simulink model "ACC_Decision_SPPVT_Integrated"  (R2024b)
settings: Solver=FixedStepAuto  StartTime=0.0  StopTime=0.05  FixedStep=0.05  RelTol=1e-3  EnableMultiTasking=on
settings Model: Creator=ZhaoY  LastModifiedBy=ZhaoY
settings SolverCC: AutoInsertRateTranBlk=on
settings DataIOCC: ExternalInput=input_data  LoadExternalInput=on

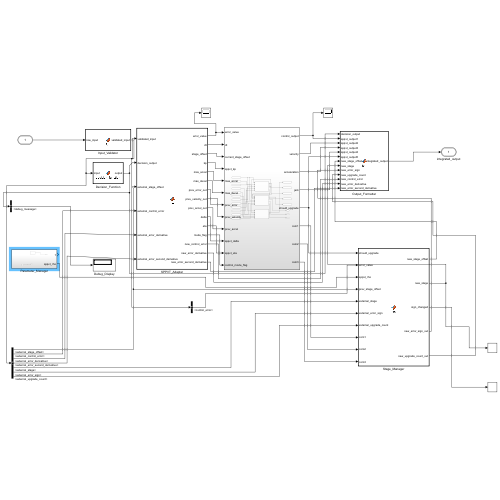
[thumbnail: Simulink's stored preview of the top-level diagram]
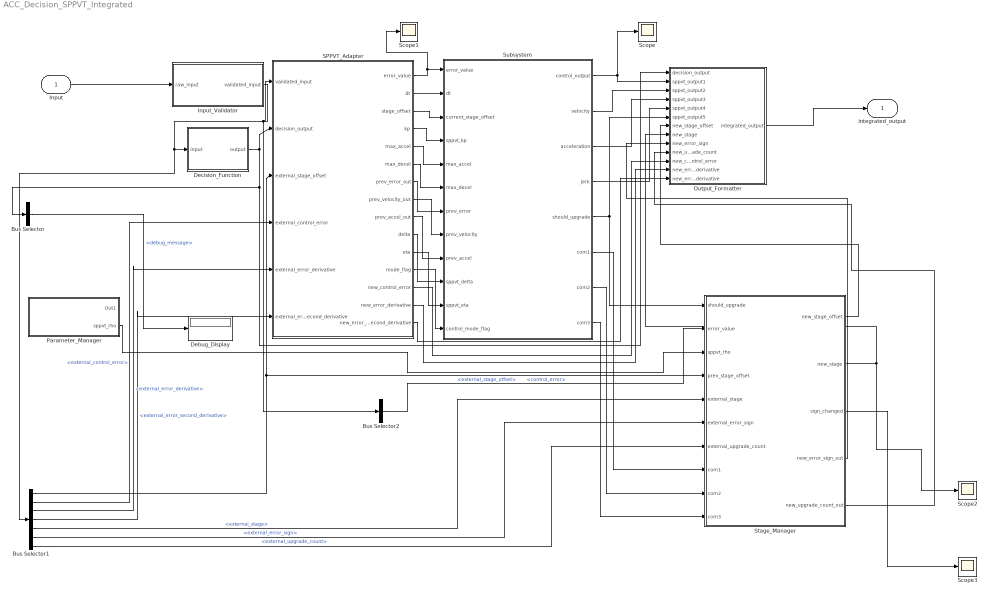
== system ACC_Decision_SPPVT_Integrated ==
  Input : Inport  OutDataTypeStr=Bus: DecisionSPPVTInputExtended  PortDimensions=1
  Bus Selector : BusSelector  OutputSignals=debug_message
  Bus Selector1 : BusSelector  OutputSignals=external_stage_offset,external_control_error,external_error_derivative,external_error_second_derivative,external_stage,external_error_sign,external_upgrade_count
  Bus Selector2 : BusSelector  OutputSignals=control_error
  Debug_Display : Display
  Decision_Function : MATLAB Function  TreatAsAtomicUnit=on
  Input_Validator : MATLAB Function  TreatAsAtomicUnit=on
  Output_Formatter : MATLAB Function  TreatAsAtomicUnit=on
  Parameter_Manager : Subsystem
  SPPVT_Adapter : MATLAB Function  TreatAsAtomicUnit=on
  Scope{,1..3} (4 alike) : Scope
  Stage_Manager : MATLAB Function  TreatAsAtomicUnit=on
  Subsystem : Subsystem
  integrated_output : Outport  OutDataTypeStr=Bus: DecisionSPPVTOutputExtended
  wires:
  Input/1 -> Input_Validator/1(raw_input)
  Input_Validator/1(validated_input) -> Bus Selector2/1, SPPVT_Adapter/1(validated_input), Bus Selector1/1, Decision_Function/1(input)
  Decision_Function/1(output) -> Output_Formatter/1(decision_output), Bus Selector/1, SPPVT_Adapter/2(decision_output)
  SPPVT_Adapter/1(error_value) -> Subsystem/1(error_value), Scope1/1
  Output_Formatter/1(integrated_output) -> integrated_output/1
  Bus Selector/1 -> Debug_Display/1  "<debug_message>"
  Stage_Manager/2(new_stage) -> Scope2/1, Output_Formatter/8(new_stage)
  Stage_Manager/3(sign_changed) -> Scope3/1
  Parameter_Manager/2(sppvt_rho) -> Stage_Manager/3(sppvt_rho)
  Bus Selector1/1 -> SPPVT_Adapter/3(external_stage_offset), Stage_Manager/4(prev_stage_offset)  "<external_stage_offset>"
  Bus Selector2/1 -> Stage_Manager/2(error_value)  "<control_error>"
  Stage_Manager/1(new_stage_offset) -> Output_Formatter/7(new_stage_offset)
  Subsystem/1(control_output) -> Output_Formatter/2(sppvt_output1), Scope/1
  Subsystem/5(should_upgrade) -> Stage_Manager/1(should_upgrade), Output_Formatter/6(sppvt_output5)
  SPPVT_Adapter/2(dt) -> Subsystem/2(dt)
  SPPVT_Adapter/3(stage_offset) -> Subsystem/3(current_stage_offset)
  SPPVT_Adapter/4(kp) -> Subsystem/4(sppvt_kp)
  SPPVT_Adapter/5(max_accel) -> Subsystem/5(max_accel)
  SPPVT_Adapter/6(max_decel) -> Subsystem/6(max_decel)
  SPPVT_Adapter/7(prev_error_out) -> Subsystem/7(prev_error)
  SPPVT_Adapter/8(prev_velocity_out) -> Subsystem/8(prev_velocity)
  SPPVT_Adapter/9(prev_accel_out) -> Subsystem/9(prev_accel)
  SPPVT_Adapter/10(delta) -> Subsystem/10(sppvt_delta)
  SPPVT_Adapter/11(eta) -> Subsystem/11(sppvt_eta)
  SPPVT_Adapter/12(mode_flag) -> Subsystem/12(control_mode_flag)
  Subsystem/2(velocity) -> Output_Formatter/3(sppvt_output2)
  Subsystem/3(acceleration) -> Output_Formatter/4(sppvt_output3)
  Subsystem/4(jerk) -> Output_Formatter/5(sppvt_output4)
  Subsystem/6(com1) -> Stage_Manager/8(com1)
  Subsystem/7(com2) -> Stage_Manager/9(com2)
  Subsystem/8(com3) -> Stage_Manager/10(com3)
  Bus Selector1/2 -> SPPVT_Adapter/4(external_control_error)  "<external_control_error>"
  Bus Selector1/3 -> SPPVT_Adapter/5(external_error_derivative)  "<external_error_derivative>"
  Bus Selector1/4 -> SPPVT_Adapter/6(external_error_second_derivative)  "<external_error_second_derivative>"
  SPPVT_Adapter/13(new_control_error) -> Output_Formatter/11(new_control_error)
  SPPVT_Adapter/14(new_error_derivative) -> Output_Formatter/12(new_error_derivative)
  SPPVT_Adapter/15(new_error_second_derivative) -> Output_Formatter/13(new_error_second_derivative)
  Bus Selector1/5 -> Stage_Manager/5(external_stage)  "<external_stage>"
  Bus Selector1/6 -> Stage_Manager/6(external_error_sign)  "<external_error_sign>"
  Bus Selector1/7 -> Stage_Manager/7(external_upgrade_count)  "<external_upgrade_count>"
  Stage_Manager/5(new_upgrade_count_out) -> Output_Formatter/10(new_upgrade_count)
  Stage_Manager/4(new_error_sign_out) -> Output_Formatter/9(new_error_sign)

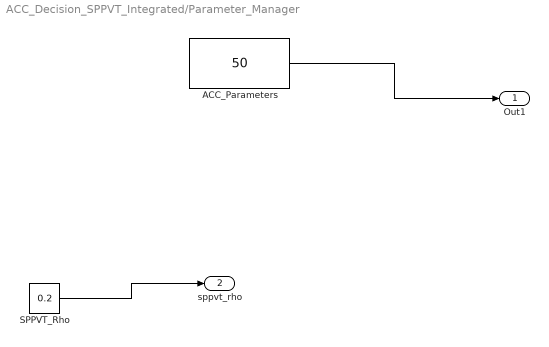
== system ACC_Decision_SPPVT_Integrated/Parameter_Manager ==
  ACC_Parameters : Constant  Value=50
  SPPVT_Rho : Constant  Value=0.2
  Out1 : Outport
  sppvt_rho : Outport  Port=2
  wires:
  ACC_Parameters/1 -> Out1/1
  SPPVT_Rho/1 -> sppvt_rho/1

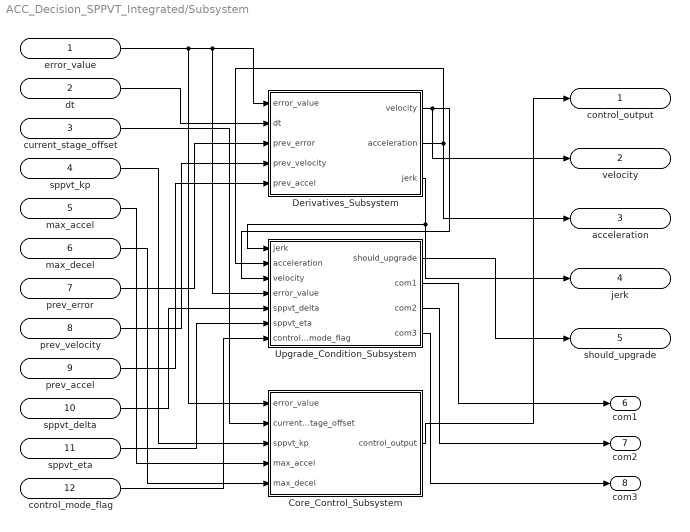
== system ACC_Decision_SPPVT_Integrated/Subsystem ==
  error_value : Inport
  dt : Inport  Port=2
  current_stage_offset : Inport  Port=3
  sppvt_kp : Inport  Port=4
  max_accel : Inport  Port=5
  max_decel : Inport  Port=6
  prev_error : Inport  Port=7
  prev_velocity : Inport  Port=8
  prev_accel : Inport  Port=9
  sppvt_delta : Inport  Port=10
  sppvt_eta : Inport  Port=11
  control_mode_flag : Inport  Port=12
  Core_Control_Subsystem : Subsystem
  Derivatives_Subsystem : Subsystem
  Upgrade_Condition_Subsystem : Subsystem
  control_output : Outport
  velocity : Outport  Port=2
  acceleration : Outport  Port=3
  jerk : Outport  Port=4
  should_upgrade : Outport  Port=5
  com1 : Outport  Port=6
  com2 : Outport  Port=7
  com3 : Outport  Port=8
  wires:
  Upgrade_Condition_Subsystem/1(should_upgrade) -> should_upgrade/1
  Derivatives_Subsystem/3(jerk) -> jerk/1, Upgrade_Condition_Subsystem/1(jerk)
  Derivatives_Subsystem/1(velocity) -> velocity/1, Upgrade_Condition_Subsystem/3(velocity)
  sppvt_eta/1 -> Upgrade_Condition_Subsystem/6(sppvt_eta)
  control_mode_flag/1 -> Upgrade_Condition_Subsystem/7(control_mode_flag)
  sppvt_delta/1 -> Upgrade_Condition_Subsystem/5(sppvt_delta)
  Derivatives_Subsystem/2(acceleration) -> acceleration/1, Upgrade_Condition_Subsystem/2(acceleration)
  Upgrade_Condition_Subsystem/2(com1) -> com1/1
  Upgrade_Condition_Subsystem/3(com2) -> com2/1
  Upgrade_Condition_Subsystem/4(com3) -> com3/1
  Core_Control_Subsystem/1(control_output) -> control_output/1
  max_decel/1 -> Core_Control_Subsystem/5(max_decel)
  max_accel/1 -> Core_Control_Subsystem/4(max_accel)
  sppvt_kp/1 -> Core_Control_Subsystem/3(sppvt_kp)
  current_stage_offset/1 -> Core_Control_Subsystem/2(current_stage_offset)
  prev_error/1 -> Derivatives_Subsystem/3(prev_error)
  prev_velocity/1 -> Derivatives_Subsystem/4(prev_velocity)
  prev_accel/1 -> Derivatives_Subsystem/5(prev_accel)
  dt/1 -> Derivatives_Subsystem/2(dt)
  error_value/1 -> Upgrade_Condition_Subsystem/4(error_value), Derivatives_Subsystem/1(error_value), Core_Control_Subsystem/1(error_value)

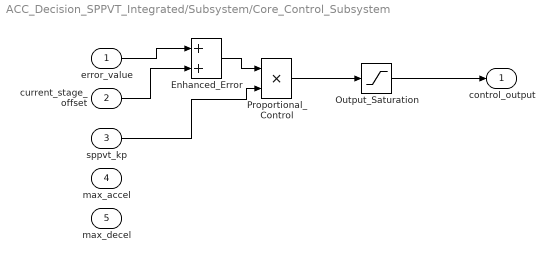
== system ACC_Decision_SPPVT_Integrated/Subsystem/Core_Control_Subsystem ==
  error_value : Inport
  current_stage_offset : Inport  Port=2
  sppvt_kp : Inport  Port=3
  max_accel : Inport  Port=4
  max_decel : Inport  Port=5
  Enhanced_Error : Sum
  Output_Saturation : Saturate  UpperLimit=2.0  LowerLimit=-3.0
  Proportional_Control : Product
  control_output : Outport
  wires:
  Proportional_Control/1 -> Output_Saturation/1
  Output_Saturation/1 -> control_output/1
  sppvt_kp/1 -> Proportional_Control/2
  current_stage_offset/1 -> Enhanced_Error/2
  error_value/1 -> Enhanced_Error/1
  Enhanced_Error/1 -> Proportional_Control/1

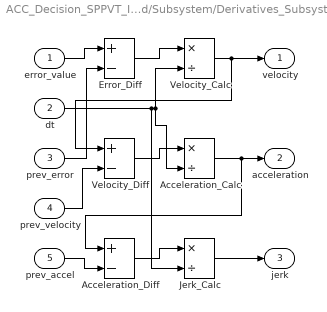
== system ACC_Decision_SPPVT_Integrated/Subsystem/Derivatives_Subsystem ==
  error_value : Inport
  dt : Inport  Port=2
  prev_error : Inport  Port=3
  prev_velocity : Inport  Port=4
  prev_accel : Inport  Port=5
  Acceleration_Calc : Product  Inputs=*/
  Acceleration_Diff : Sum  Inputs=+-
  Error_Diff : Sum  Inputs=+-
  Jerk_Calc : Product  Inputs=*/
  Velocity_Calc : Product  Inputs=*/
  Velocity_Diff : Sum  Inputs=+-
  velocity : Outport
  acceleration : Outport  Port=2
  jerk : Outport  Port=3
  wires:
  Velocity_Calc/1 -> Velocity_Diff/1, velocity/1
  Acceleration_Calc/1 -> Acceleration_Diff/1, acceleration/1
  Jerk_Calc/1 -> jerk/1
  error_value/1 -> Error_Diff/1
  prev_error/1 -> Error_Diff/2
  Error_Diff/1 -> Velocity_Calc/1
  prev_accel/1 -> Acceleration_Diff/2
  prev_velocity/1 -> Velocity_Diff/2
  Acceleration_Diff/1 -> Jerk_Calc/1
  dt/1 -> Jerk_Calc/2, Acceleration_Calc/2, Velocity_Calc/2
  Velocity_Diff/1 -> Acceleration_Calc/1

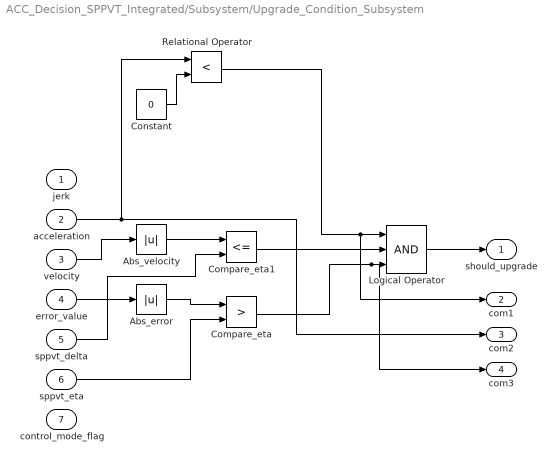
== system ACC_Decision_SPPVT_Integrated/Subsystem/Upgrade_Condition_Subsystem ==
  jerk : Inport
  acceleration : Inport  Port=2
  velocity : Inport  Port=3
  error_value : Inport  Port=4
  sppvt_delta : Inport  Port=5
  sppvt_eta : Inport  Port=6
  control_mode_flag : Inport  Port=7
  Abs_error : Abs  SaturateOnIntegerOverflow=off
  Abs_velocity : Abs  SaturateOnIntegerOverflow=off
  Compare_eta : RelationalOperator  Operator=>  OutDataTypeStr=boolean  RndMeth=Simplest  InputSameDT=off
  Compare_eta1 : RelationalOperator  Operator=<=  OutDataTypeStr=boolean  RndMeth=Simplest  InputSameDT=off
  Constant : Constant  Value=0
  Logical Operator : Logic  Inputs=3  AllPortsSameDT=off  OutDataTypeStr=boolean
  Relational Operator : RelationalOperator  Operator=<  OutDataTypeStr=boolean  RndMeth=Simplest  InputSameDT=off
  should_upgrade : Outport
  com1 : Outport  Port=2
  com2 : Outport  Port=3
  com3 : Outport  Port=4
  wires:
  error_value/1 -> Abs_error/1
  Abs_error/1 -> Compare_eta/1
  sppvt_eta/1 -> Compare_eta/2
  acceleration/1 -> com2/1, Relational Operator/1
  Constant/1 -> Relational Operator/2
  velocity/1 -> Abs_velocity/1
  Abs_velocity/1 -> Compare_eta1/1
  sppvt_delta/1 -> Compare_eta1/2
  Relational Operator/1 -> com1/1, Logical Operator/1
  Compare_eta1/1 -> Logical Operator/2
  Compare_eta/1 -> com3/1, Logical Operator/3
  Logical Operator/1 -> should_upgrade/1

== matlab function ACC_Decision_SPPVT_Integrated/Stage_Manager ==
  data: new_stage_offset output; should_upgrade input; new_stage output; sign_changed output; new_error_sign_out output; error_value input; sppvt_rho input; prev_stage_offset input; external_stage input; external_error_sign input; external_upgrade_count input; com1 input; com2 input; com3 input; new_upgrade_count_out output
  function [new_stage_offset, new_stage, sign_changed, new_error_sign_out, new_upgrade_count_out] = fcn(should_upgrade, error_value, sppvt_rho, prev_stage_offset, external_stage, external_error_sign, external_upgrade_count, com1, com2, com3)
  %#codegen
  % Stateless SPPVT Stage Manager with scalar-based state management
  % Compatible with 21/22-field bus design (all scalar version)

  % Extract states from input scalars (replaces persistent variables and array extraction)
  current_stage = int32(external_stage);
  prev_error_sign = int32(external_error_sign);
  upgrade_count = int32(external_upgrade_count);

  current_stage_offset = prev_stage_offset;

  % Calculate current error sign
  if abs(error_value) < 1e-6
      current_sign = int32(0);     % Near zero
  elseif error_value > 0
      current_sign = int32(1);     % Positive error
  else
      current_sign = int32(-1);    % Negative error
  end

  % Initialize outputs with current values
  new_stage = current_stage;
  sign_changed = false;

  % Error sign change detection
  if (prev_error_sign ~= 0) && (current_sign ~= 0) && (prev_error_sign ~= current_sign)
      % Sign change: reset to initial stage
      sign_changed = true;

      % Reset all states to initial level
      new_stage = int32(1);
      new_stage_offset = 0.0;      % Initial stage offset is 0
      upgrade_count = int32(0);

  elseif should_upgrade && ~sign_changed
      % No sign change and upgrade condition met
      new_stage = new_stage + int32(1);
      upgrade_count = upgrade_count + int32(1);

      % Calculate new stage offset based on error sign (consistent with existing logic)
      if error_value > 0
          % Positive error: increase positive stage offset
          new_stage_offset = prev_stage_offset + sppvt_rho * abs(error_value);
      else
          % Negative error: increase negative stage offset
          new_stage_offset = prev_stage_offset - sppvt_rho * abs(error_value);
      end

      % Limit stage offset range [-100, 100] to prevent infinite accumulation
      new_stage_offset = max(-100.0, min(100.0, new_stage_offset));

  else
      % No upgrade: maintain current state
      new_stage_offset = prev_stage_offset;
  end

  % Update error sign history (only for non-zero errors)
  new_error_sign = prev_error_sign;
  if current_sign ~= 0
      new_error_sign = current_sign;
  end

  % Output individual scalars for next cycle (to be captured by Python)
  % Scalar outputs: new_error_sign_out, new_upgrade_count_out (new_stage already in output list)
  new_error_sign_out = double(new_error_sign);
  new_upgrade_count_out = double(upgrade_count);

  % Print the three conditional variables using fprintf
  % Print the three conditional variables as 'true' or 'false' with detailed labels
  fprintf('Condition 1 (com1): %s\n', string(com1));
  fprintf('Condition 2 (com2): %f\n', double(com2));
  fprintf('Condition 3 (com3): %s\n', string(com3));
  end

== matlab function ACC_Decision_SPPVT_Integrated/Decision_Function ==
  data: input input Bus: DecisionSPPVTInputExtended; output output Bus: DecisionSPPVTOutputExtended
function output = decision_function(input)
%DECISION_FUNCTION ACC决策状态机的MATLAB实现
%   适用于MATLAB 2024b，在Simulink中作为MATLAB Function块使用
%   
%   输入: DecisionSPPVTInput总线
%   输出: 决策相关的输出结构
%
%   状态定义 (根据decision.md和acc_decision.py):
%   S0 = 0: 在控状态 (ACTIVE_CONTROL)
%   S1 = 1: 适速有史待命 (ADAPTIVE_HISTORY_STANDBY)  
% %   S2 = 2: 适速无史待命 (ADAPTIVE_NO_HISTORY_STANDBY)
%   S3 = 3: 低速状态 (LOW_SPEED)
%
%   决策定义:
%   R1 = 1: 速度降低 (DECREASE_SPEED)
%   R2 = 2: 速度增加 (INCREASE_SPEED)
%   R3 = 3: 时距降低 (DECREASE_DISTANCE)
%   R4 = 4: 时距增加 (INCREASE_DISTANCE)
%   R5 = 5: 无继控制 (ACTIVATE_CURRENT_SPEED)
%   R6 = 6: 继承控制 (ACTIVATE_INHERITED_SPEED)
%   R7 = 7: 扭矩仲裁 (TORQUE_ARBITRATION)
%   R8 = 8: 系统待命 (SYSTEM_STANDBY)

% 保留必要的persistent变量（仅用于调试计数）
persistent debug_counter

% 初始化调试计数器
if isempty(debug_counter)
    debug_counter = int32(0);
end

% 提取输入参数
ego_speed_kmh = input.ego_speed_kmh;
% ego_speed_ms = input.ego_speed_ms;          % 未使用，决策逻辑只需要km/h
command_type = input.command_type;
command_active = input.command_active;
manual_throttle_active = input.manual_throttle_active;
% control_error = input.control_error;        % 决策模块不直接使用控制误差
% control_mode_flag = input.control_mode_flag; % 决策模块不直接使用模式标志
input_V_target_kmh = input.V_target_kmh;
input_V_min_kmh = input.V_min_kmh;
input_G2_s = input.G2_s;
% timestamp = input.timestamp;                % 决策逻辑不需要时间戳

% 更新参数
V_target_kmh = input_V_target_kmh;
V_min_kmh = input_V_min_kmh;
G2_s = input_G2_s;

%% 键盘参数修改逻辑 (在状态机逻辑之前处理)
if command_active
    speed_step = 5.0;  % 速度调整步长 (km/h)
    time_gap_step = 0.2; % 时距调整步长 (s)

    switch command_type
        case 1 % I0: Decrease speed -> E key
            V_target_kmh = max(V_min_kmh, V_target_kmh - speed_step);
            fprintf('Keyboard: E key decrease speed, V_target: %.1f km/h\n', V_target_kmh);

        case 2 % I1: Increase speed -> Q key
            V_target_kmh = min(120.0, V_target_kmh + speed_step);
            fprintf('Keyboard: Q key increase speed, V_target: %.1f km/h\n', V_target_kmh);

        case 3 % I2: Decrease time gap -> T key
            G2_s = max(1.0, G2_s - time_gap_step);
            fprintf('Keyboard: T key decrease gap, G2: %.1f s\n', G2_s);

        case 4 % I3: Increase time gap -> R key
            G2_s = min(5.0, G2_s + time_gap_step);
            fprintf('Keyboard: R key increase gap, G2: %.1f s\n', G2_s);

        case 7 % I6: Cancel ACC -> C key
            fprintf('Keyboard: C key cancel ACC\n');
            % 取消逻辑在状态机中处理
    end
end

% 增加调试计数器
debug_counter = debug_counter + 1;

%% 从输入获取决策状态信息（替代persistent变量）
% 如果总线中没有这些字段，使用默认值
if isfield(input, 'current_state')
    current_state = input.current_state;
else
    current_state = int32(2); % 默认S2状态
end

if isfield(input, 'has_history')
    has_history = input.has_history;
else
    has_history = false; % 默认无历史
end

if isfield(input, 'last_active_decision')
    last_active_decision = input.last_active_decision;
else
    last_active_decision = int32(8); % 默认R8
end

%% 获取SPPVT状态外化字段（虽然决策模块不直接使用，但需要传递）
% 这些字段将在输出中保持原值，由SPPVT模块使用
if isfield(input, 'external_stage_offset')
    external_stage_offset = input.external_stage_offset;
else
    external_stage_offset = 0.0; % 默认级差
end

if isfield(input, 'external_stage')
    external_stage = input.external_stage;
else
    external_stage = 1.0; % 默认阶段
end

if isfield(input, 'external_error_sign')
    external_error_sign = input.external_error_sign;
else
    external_error_sign = 0.0; % 默认误差符号
end

if isfield(input, 'external_upgrade_count')
    external_upgrade_count = input.external_upgrade_count;
else
    external_upgrade_count = 0.0; % 默认升级计数
end

if isfield(input, 'external_control_error')
    external_control_error = input.external_control_error;
else
    external_control_error = 0.0; % 默认控制误差
end

if isfield(input, 'external_error_derivative')
    external_error_derivative = input.external_error_derivative;
else
    external_error_derivative = 0.0; % 默认控制误差导数
end

if isfield(input, 'external_error_second_derivative')
    external_error_second_derivative = input.external_error_second_derivative;
else
    external_error_second_derivative = 0.0; % 默认控制误差二阶导数
end

%% 状态机主逻辑 - 使用next_state管理状态转移
next_state = current_state; % 默认保持当前状态
next_has_history = has_history; % 默认保持历史状态
next_last_active_decision = last_active_decision; % 默认保持决策
torque_arbitration_active = false;

% 基于当前状态设置默认决策
if current_state == 0
    control_enabled = true;
    current_decision = last_active_decision; % 使用上次有效决策实现持续性
    % 如果历史决策无效，提供后备值
    if ~(current_decision >= 1 && current_decision <= 7)
        current_decision = int32(5); % 默认 R5: 无继控制
    end
else
    control_enabled = false;
    current_decision = int32(8); % R8: 系统待命
end

% 基于车速的自动状态转移
if ego_speed_kmh < V_min_kmh
    if current_state ~= 3
        next_state = int32(3); % 转移到S3: 低速状态
        control_enabled = false;
        current_decision = int32(8);
    end
else
    % 从S3状态恢复
    if current_state == 3
        if has_history
            next_state = int32(1); % 恢复到S1: 有史待命
        else
            next_state = int32(2); % 恢复到S2: 无史待命
        end
        control_enabled = false;
        current_decision = int32(8);
    end
end

% 处理激活的指令
if command_active
    switch current_state
        case 0 % S0: 在控状态
            [next_state, current_decision, control_enabled, torque_arbitration_active] = ...
                handle_active_control_state(command_type, ego_speed_kmh, manual_throttle_active, V_target_kmh, G2_s);

        case 1 % S1: 适速有史待命
            [next_state, current_decision, control_enabled, next_has_history, V_target_kmh, G2_s] = ...
                handle_adaptive_history_standby_state(command_type, ego_speed_kmh, V_target_kmh, G2_s, input_V_target_kmh, input_G2_s);

        case 2 % S2: 适速无史待命
            [next_state, current_decision, control_enabled, next_has_history, V_target_kmh, G2_s] = ...
                handle_adaptive_no_history_standby_state(command_type, ego_speed_kmh, input_V_target_kmh, input_G2_s);

        case 3 % S3: 低速状态
            % 低速状态下，指令不进入控制
            current_decision = int32(8);
            control_enabled = false;

        otherwise
            % 错误状态，重置到无史待命
            next_state = int32(2);
            current_decision = int32(8);
            control_enabled = false;
            next_has_history = false;
    end
end

% 更新有效决策用于持续性控制
if current_decision >= 1 && current_decision <= 7
    next_last_active_decision = current_decision;
end

%% 计算调试信息值（在赋值前准备）
control_flag = int32(control_enabled);
if mod(debug_counter, 20) == 0 % 每20个周期输出一次调试信息
    % 调试代码: 1000 + 状态*100 + 决策*10 + 控制使能标志
    debug_code = int32(1000 + current_state*100 + current_decision*10 + control_flag);
    debug_message_value = debug_code;

    % 添加MATLAB Function调试输出
    fprintf('Decision Function Debug: State=%d->%d, Decision=%d, Control=%d, Active=%d, Cmd=%d, DebugCode=%d\n', ...
            current_state, next_state, current_decision, int32(control_enabled), int32(command_active), command_type, debug_code);
else
    % 非调试周期显示简单计数器
    debug_message_value = debug_counter;
end

%% 构造输出 - 严格按照DecisionSPPVTOutputExtended总线定义顺序赋值所有22个字段
output = struct();

% 1-6: 来自决策系统的基本信息
output.control_enabled = logical(control_enabled);
output.current_state = int32(next_state);  % 修正：输出当前步计算的实际状态
output.current_decision = int32(current_decision);
output.torque_arbitration_active = logical(torque_arbitration_active);
output.updated_V_target_kmh = double(V_target_kmh);
output.updated_G2_s = double(G2_s);

% 7-11: SPPVT相关字段的默认值（这些将由后续模块填充）
output.sppvt_control_output = 0.0;
output.sppvt_velocity_output = 0.0;
output.sppvt_acceleration_output = 0.0;
output.sppvt_stage_output = 0.0;
output.sppvt_status_output = 0.0;

% 12: 调试信息
output.debug_message = debug_message_value;

% 13-15: 决策状态输出字段（状态外化支持）
output.next_state = int32(next_state);
output.next_has_history = logical(next_has_history);
output.next_last_active_decision = int32(next_last_active_decision);

% 16-22: SPPVT状态输出字段（传递外部输入，由后续SPPVT模块更新）- 全部标量化
output.new_stage_offset = double(external_stage_offset);
output.new_stage = double(external_stage);
output.new_error_sign = double(external_error_sign);
output.new_upgrade_count = double(external_upgrade_count);
output.new_control_error = double(external_control_error);
output.new_error_derivative = double(external_error_derivative);
output.new_error_second_derivative = double(external_error_second_derivative);

end

%% 状态处理函数

function [new_state, decision, control_enabled, torque_arbitration] = ...
    handle_active_control_state(command_type, ego_speed_kmh, manual_throttle_active, V_target_kmh, G2_s)
%处理在控状态 S0 (根据decision.md)

new_state = int32(0); % 默认保持在控状态
control_enabled = true;
torque_arbitration = false;

% 初始化所有输出变量（确保在所有执行路径上都有定义）
decision = int32(8); % 默认系统待命

switch command_type
    case 1 % I0: 降速指令
        decision = int32(1); % R1: 速度降低
        
    case 2 % I1: 增速指令
        decision = int32(2); % R2: 速度增加
        
    case 3 % I2: 降距指令
        decision = int32(3); % R3: 时距降低
        
    case 4 % I3: 增距指令
        decision = int32(4); % R4: 时距增加
        
    case 5 % I4: 油门指令
        decision = int32(7); % R7: 扭矩仲裁
        torque_arbitration = true;
        % 状态保持S0，但控制权可能被驾驶员超越
        
    case 6 % I5: 刹车指令
        new_state = int32(1); % 转到S1: 适速有史待命
        decision = int32(8); % R8: 系统待命
        control_enabled = false;
        
    case 7 % I6: 取消ACC指令
        new_state = int32(1); % 转到S1: 适速有史待命
        decision = int32(8); % R8: 系统待命
        control_enabled = false;
        
    otherwise
        decision = int32(8); % R8: 系统待命
end
end

function [new_state, decision, control_enabled, has_history, V_target_kmh, G2_s] = ...
    handle_adaptive_history_standby_state(command_type, ego_speed_kmh, current_V_target, current_G2, input_V_target, input_G2)
%处理适速有史待命状态 S1 (根据decision.md)

new_state = int32(1); % 默认保持S1状态
control_enabled = false;
has_history = true; % 保持历史数据

% 初始化所有输出变量（确保在所有执行路径上都有定义）
V_target_kmh = current_V_target;
G2_s = current_G2;
decision = int32(8); % 默认系统待命

switch command_type
    case 1 % I0: 降速指令
        new_state = int32(0); % 转到S0: 在控状态
        decision = int32(5); % R5: 无继控制 (当速启控)
        control_enabled = true;
        V_target_kmh = input_V_target; % 使用当前速度作为目标
        G2_s = input_G2;
        
    case 2 % I1: 增速指令
        new_state = int32(0); % 转到S0: 在控状态
        decision = int32(6); % R6: 继承控制 (使用历史速度)
        control_enabled = true;
        % V_target_kmh和G2_s保持历史值不变
        
    otherwise % I2-I6: 其他指令
        decision = int32(8); % R8: 系统待命
        % 状态保持S1，参数保持历史值
end
end

function [new_state, decision, control_enabled, has_history, V_target_kmh, G2_s] = ...
    handle_adaptive_no_history_standby_state(command_type, ego_speed_kmh, input_V_target, input_G2)
%处理适速无史待命状态 S2 (根据decision.md)

new_state = int32(2); % 默认保持S2状态
control_enabled = false;
has_history = false; % 仍然无历史数据

% 初始化所有输出变量（确保在所有执行路径上都有定义）
V_target_kmh = input_V_target;
G2_s = input_G2;
decision = int32(8); % 默认系统待命

switch command_type
    case 1 % I0: 降速指令
        new_state = int32(0); % 转到S0: 在控状态
        decision = int32(5); % R5: 无继控制 (当速启控)
        control_enabled = true;
        has_history = true; % 启控后产生历史数据
        V_target_kmh = input_V_target; % 使用当前速度作为目标
        G2_s = input_G2;
        
    otherwise % I1-I6: 其他指令
        decision = int32(8); % R8: 系统待命
        % 状态保持S2，无历史数据
        % V_target_kmh和G2_s已在函数开头初始化
end
end

== matlab function ACC_Decision_SPPVT_Integrated/Input_Validator ==
  data: raw_input input Bus: DecisionSPPVTInputExtended; validated_input output Bus: DecisionSPPVTInputExtended
function validated_input = fcn(raw_input)
%#codegen
%
% 输入验证和预处理
% 输入: raw_input (DecisionSPPVTInput总线)
% 输出: validated_input (经过验证和修正的总线)

validated_input = raw_input;

% 接下来，在输出变量上执行数值范围检查，防止异常值进入下游模块。
validated_input.ego_speed_kmh = max(0, min(200, raw_input.ego_speed_kmh));
validated_input.ego_speed_ms = max(0, min(60, raw_input.ego_speed_ms));
validated_input.V_target_kmh = max(30, min(120, raw_input.V_target_kmh));
validated_input.V_min_kmh = max(20, min(50, raw_input.V_min_kmh));
validated_input.G2_s = max(1.0, min(8.0, raw_input.G2_s));


% 确保最低车速始终小于或等于目标车速。
if validated_input.V_min_kmh > validated_input.V_target_kmh
    validated_input.V_min_kmh = validated_input.V_target_kmh - 10;
end

% 时间戳直接透传
validated_input.timestamp = raw_input.timestamp;

end

== matlab function ACC_Decision_SPPVT_Integrated/Output_Formatter ==
  data: decision_output input; integrated_output output Bus: DecisionSPPVTOutputExtended; sppvt_output1 input; sppvt_output2 input; sppvt_output3 input; sppvt_output4 input; sppvt_output5 input; new_stage_offset input; new_stage input; new_error_sign input; new_upgrade_count input; new_control_error input; new_error_derivative input; new_error_second_derivative input
function integrated_output = fcn(decision_output, sppvt_output1, sppvt_output2, sppvt_output3, sppvt_output4, sppvt_output5, new_stage_offset, new_stage, new_error_sign, new_upgrade_count, new_control_error, new_error_derivative, new_error_second_derivative)
%#codegen
% Output_Formatter - 21/22-field state externalization version (all scalar)
% Integrates decision, SPPVT output and state output for Python state capture
%
% Inputs:
%   decision_output - DecisionSPPVTOutput from Decision_Function (includes next_state and other decision state output fields)
%   sppvt_output1-5 - 5 outputs from SPPVT_Control (control, velocity, acceleration, jerk, status)
%   new_stage_offset - Stage offset (scalar)
%   new_stage - Stage Manager new stage (scalar)
%   new_error_sign - Stage Manager new error sign (scalar)
%   new_upgrade_count - Stage Manager new upgrade count (scalar)
%   new_control_error - New control error (scalar)
%   new_error_derivative - New control error derivative (scalar)
%   new_error_second_derivative - New control error second derivative (scalar)
%
% Output: integrated_output - DecisionSPPVTOutputExtended (22 fields)

%% 构造集成输出结构
integrated_output = struct();

%% 按照总线定义顺序赋值所有字段（确保代码生成兼容性）
% 根据DecisionSPPVTOutputExtended总线定义的22字段顺序

% 1-6: 来自决策系统的信息
integrated_output.control_enabled = decision_output.control_enabled;
integrated_output.current_state = decision_output.current_state;
integrated_output.current_decision = decision_output.current_decision;
integrated_output.torque_arbitration_active = decision_output.torque_arbitration_active;
integrated_output.updated_V_target_kmh = decision_output.updated_V_target_kmh;
integrated_output.updated_G2_s = decision_output.updated_G2_s;

% 7-11: SPPVT controller outputs (double precision)
integrated_output.sppvt_control_output = double(sppvt_output1);
integrated_output.sppvt_velocity_output = double(sppvt_output2);
integrated_output.sppvt_acceleration_output = double(sppvt_output3);
% 注意：sppvt_output4是jerk，不是stage，stage来自Stage_Manager
integrated_output.sppvt_stage_output = double(new_stage);  % 从Stage_Manager获取stage值（标量）
integrated_output.sppvt_status_output = double(sppvt_output5);

% 12: Debug information (composite code)
debug_code = int32(3000 + decision_output.current_state*100 + ...
                 mod(int32(sppvt_output5), 10)*10 + ...
                 int32(decision_output.control_enabled));
integrated_output.debug_message = debug_code;

% 13-15: Decision module state outputs
integrated_output.next_state = decision_output.next_state;
integrated_output.next_has_history = decision_output.next_has_history;
integrated_output.next_last_active_decision = decision_output.next_last_active_decision;

% 16-22: SPPVT state outputs consumed in Python (全部标量化)

% 16: Stage offset (scalar)
integrated_output.new_stage_offset = double(new_stage_offset);

% 17-19: Stage Manager states (全部标量)
integrated_output.new_stage = double(new_stage);
integrated_output.new_error_sign = double(new_error_sign);
integrated_output.new_upgrade_count = double(new_upgrade_count);

% 20-22: Adapter states - 控制误差及其导数 (全部标量)
% 修正：用SPPVT实际计算的导数值替换Adapter传来的占位值
integrated_output.new_control_error = double(new_control_error);
integrated_output.new_error_derivative = double(sppvt_output2);  % 误差的一阶导数 (velocity)
integrated_output.new_error_second_derivative = double(sppvt_output3);  % 误差的二阶导数 (acceleration)

% 调试输出（22字段版本，包含完整状态外化信息）
if mod(decision_output.debug_message, 50) == 0
    fprintf("Output_Formatter Input: State=%d, Decision=%d, Control=%d, Debug=%d\n", ...
            int32(decision_output.current_state), int32(decision_output.current_decision), ...
            int32(decision_output.control_enabled), int32(decision_output.debug_message));
    fprintf("Integrated Output: State=S%d->S%d, Decision=R%d, Control=%d, SPPVT=%.3f\n", ...
            int32(decision_output.current_state), int32(decision_output.next_state), ...
            int32(decision_output.current_decision), int32(decision_output.control_enabled), double(sppvt_output1));

    % 决策状态外化调试输出
    fprintf("Decision State: next_state=S%d, next_history=%d, next_decision=R%d\n", ...
            int32(decision_output.next_state), int32(decision_output.next_has_history), ...
            int32(decision_output.next_last_active_decision));

    % SPPVT状态外化调试输出（标量版本）
    fprintf("SPPVT State: StageOffset=%.3f, Stage=%.0f, ErrorSign=%.0f, UpgradeCount=%.0f\n", ...
            double(new_stage_offset), double(new_stage), double(new_error_sign), double(new_upgrade_count));
    fprintf("Error States: ControlError=%.3f, Derivative=%.3f, SecondDerivative=%.3f\n", ...
            double(new_control_error), double(sppvt_output2), double(sppvt_output3));
end

end

== matlab function ACC_Decision_SPPVT_Integrated/SPPVT_Adapter ==
  data: validated_input input; decision_output input; error_value output; dt output; stage_offset output; kp output; max_accel output; max_decel output; prev_error_out output; prev_velocity_out output; prev_accel_out output; delta output; eta output; mode_flag output; external_stage_offset input; external_control_error input; new_control_error output double; external_error_derivative input; external_error_second_derivative input; new_error_derivative output; new_error_second_derivative output
function [error_value, dt, stage_offset, kp, max_accel, max_decel, prev_error_out, prev_velocity_out, prev_accel_out, delta, eta, mode_flag, new_control_error, new_error_derivative, new_error_second_derivative] = fcn(validated_input, decision_output, external_stage_offset, external_control_error, external_error_derivative, external_error_second_derivative)
%#codegen
% SPPVT接口适配器 - 支持外部状态注入版本 (全部标量化)
% 输入:
%   validated_input - 验证后的输入总线
%   decision_output - 决策输出总线
%   external_stage_offset - 外部级差状态
%   external_control_error - 外部控制误差
%   external_error_derivative - 外部控制误差的导数
%   external_error_second_derivative - 外部控制误差的二阶导数
% 输出:
%   1-12: 12个独立信号匹配sppvt_control_model的12个输入端口
%   13-15: 新的误差状态（标量化）- new_control_error, new_error_derivative, new_error_second_derivative

%% 直接使用外部状态（从Bus Selector传入）- 全部标量化
current_stage_offset = external_stage_offset;

% 直接使用输入的标量参数（不再需要从数组提取）
% 注意：velocity和accel实际上是误差的一阶和二阶导数
prev_error = external_control_error;
prev_velocity = external_error_derivative;           % 控制误差的一阶导数
prev_accel = external_error_second_derivative;       % 控制误差的二阶导数

%% 根据决策结果确定控制误差
if decision_output.control_enabled
    % 控制激活时使用实际误差
    error_value = validated_input.control_error;
else
    % 控制未激活时误差为0
    error_value = 0.0;
end

%% 分配12个独立输出信号
dt = 0.05;                                      % [2] dt 时间步长 (硬编码为50ms)
stage_offset = current_stage_offset;            % [3] 当前级差 (状态变量)
kp = 1.0;                                       % [4] sppvt_kp 比例系数 (硬编码)
max_accel = 2.0;                                % [5] max_accel 最大加速度 (硬编码)
max_decel = -3.0;                               % [6] max_decel 最大减速度 (硬编码)
prev_error_out = prev_error;                    % [7] 上次误差 (状态变量)
prev_velocity_out = prev_velocity;              % [8] 上次速度 (状态变量)
prev_accel_out = prev_accel;                    % [9] 上次加速度 (状态变量)
delta = 0.05;                                   % [10] sppvt_delta 控制参数 
eta = 0.5;                                      % [11] sppvt_eta 控制参数 
mode_flag = double(validated_input.control_mode_flag); % [12] 控制模式标志

%% 输出新的误差状态（第13-15个输出）- 全部标量化
% 用于Output_Formatter的误差状态字段
% 注意：这些是当前计算的误差值，导数将由SPPVT模块计算
new_control_error = error_value;
new_error_derivative = external_error_derivative;  % 保持输入值，将由SPPVT更新
new_error_second_derivative = external_error_second_derivative;  % 保持输入值，将由SPPVT更新

% 调试输出 - 显示关键参数
if abs(error_value) > 0.01
    fprintf("SPPVT Adapter: Error=%.3f, Speed=%.3f, Stage=%.3f, PrevError=%.3f, Mode=%d, Control=%d\n", ...
            error_value, validated_input.ego_speed_ms, current_stage_offset, prev_error, ...
            int32(validated_input.control_mode_flag), int32(decision_output.control_enabled));
end
end
